simulink model "exp3"  (R2025b)
settings: Solver=VariableStepAuto  StartTime=0.0  StopTime=10.0  RelTol=1e-3
settings Model: Creator=SUBHASH  LastModifiedBy=SUBHASH

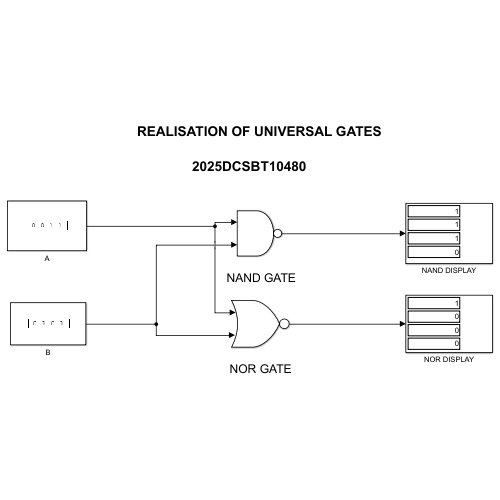
[thumbnail: Simulink's stored preview of the top-level diagram]
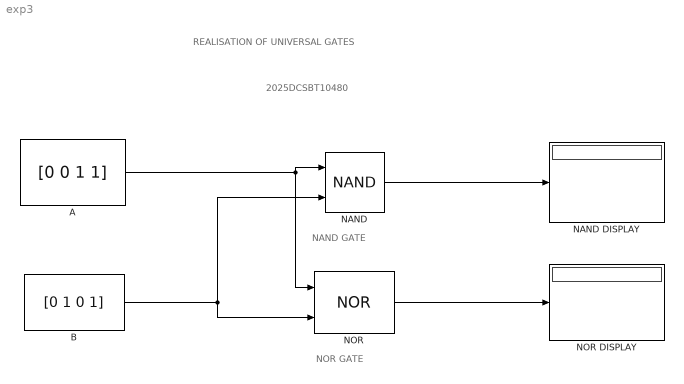
== system exp3 ==
  note: 2025DCSBT10480
  note: REALISATION OF UNIVERSAL GATES
  note: NOR GATE
  note: NAND GATE
  A : Constant  Value=[0 0 1 1]
  B : Constant  Value=[0 1 0 1]
  NAND : Logic  Operator=NAND  IconShape=distinctive  AllPortsSameDT=off  OutDataTypeStr=boolean
  NAND DISPLAY : Display
  NOR : Logic  Operator=NOR  IconShape=distinctive  AllPortsSameDT=off  OutDataTypeStr=boolean
  NOR DISPLAY : Display
  wires:
  A/1 -> NOR/1, NAND/1
  B/1 -> NAND/2, NOR/2
  NAND/1 -> NAND DISPLAY/1
  NOR/1 -> NOR DISPLAY/1
